simulink model "Lidar_System_CheckZero"  (Simulink 7.5)
settings: Solver=FixedStepDiscrete  StartTime=0.0  StopTime=inf  FixedStep=0.1  MaxStep=0.2  RelTol=1e-3
settings Model: Creator=gclayton  LastModifiedBy=wildcat
settings DebuggingCC: InheritedTsInSrcMsg=none  StrictBusMsg=Warning
settings RTWCC: SystemTargetFile=rlnx.tlc  GenCodeOnly=on  TemplateMakefile=rlnx_ubuntu.tmf  Description=Linux Real-Time Target  ProcessScript=rlnx_make_rtw_hook
settings RTWCC: CustomInclude=|
  | /usr/local/include/opencv/
  | /usr/local/include/
settings CodeAppCC: GenerateComments=off  SimulinkBlockComments=off
settings STFCustomTargetCC: ModelReferenceCompliant=off  GeneratePreprocessorConditionals=Disable all  MatFileLogging=on  SystemTargetFile=rlnx.tlc
settings GRTTargetCC: ModelReferenceCompliant=off  ParMdlRefBuildCompliant=off  CompOptLevelCompliant=off  ExtModeMexFile=noextcomm
settings CustomProperty: DataType=string  Value="-lm -ldl /usr/local/lib/libopencv_highgui.so.2.4 /usr/local/lib/libopencv_core.so.2.4 /usr/local/lib/libopencv_imgproc.so.2.4  -lc_urg -lc_urg_connection -lc_urg_system -lphidget21 -llcm"
settings EnumStrPairs: String=PC

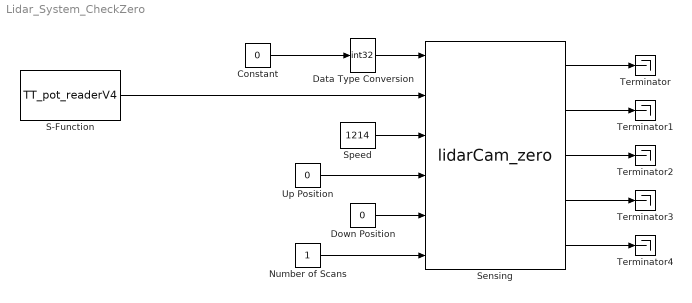
== system Lidar_System_CheckZero ==
  Constant : Constant  Value=0  OutDataType=fixdt(1, 16)  OutScaling=2^0
  Data Type Conversion : DataTypeConversion  OutDataTypeMode=int32  OutDataType=fixdt(1, 16)  OutScaling=2^0  OutDataTypeStr=int32
  Down Position : Constant  Value=0  OutDataType=fixdt(1, 16)  OutScaling=2^0
  Number of Scans : Constant  OutDataType=fixdt(1, 16)  OutScaling=2^0
  S-Function : S-Function  FunctionName=TT_pot_readerV4  EnableBusSupport=off
  Sensing : S-Function  FunctionName=lidarCam_zero  EnableBusSupport=off
  Speed : Constant  Value=1214  OutDataType=fixdt(1, 16)  OutScaling=2^0
  Terminator{,1..4} (5 alike) : Terminator
  Up Position : Constant  Value=0  OutDataType=fixdt(1, 16)  OutScaling=2^0
  wires:
  S-Function/1 -> Sensing/2
  Data Type Conversion/1 -> Sensing/1
  Constant/1 -> Data Type Conversion/1
  Speed/1 -> Sensing/3
  Up Position/1 -> Sensing/4
  Down Position/1 -> Sensing/5
  Number of Scans/1 -> Sensing/6
  Sensing/1 -> Terminator/1
  Sensing/2 -> Terminator1/1
  Sensing/3 -> Terminator2/1
  Sensing/4 -> Terminator3/1
  Sensing/5 -> Terminator4/1
